simulink model "QuadSim"  (R2015a)
settings: Solver=ode45  StartTime=0.0  StopTime=10.0  RelTol=1e-3
undefined symbols (not defined in the file or in its folder): magnitude
libraries: aerolibutil x67, dspmathops x4, simulink_extras x2, dspinverses x1
(part 1 of 2)
settings Model: Creator=Nick  LastModifiedBy=Nick

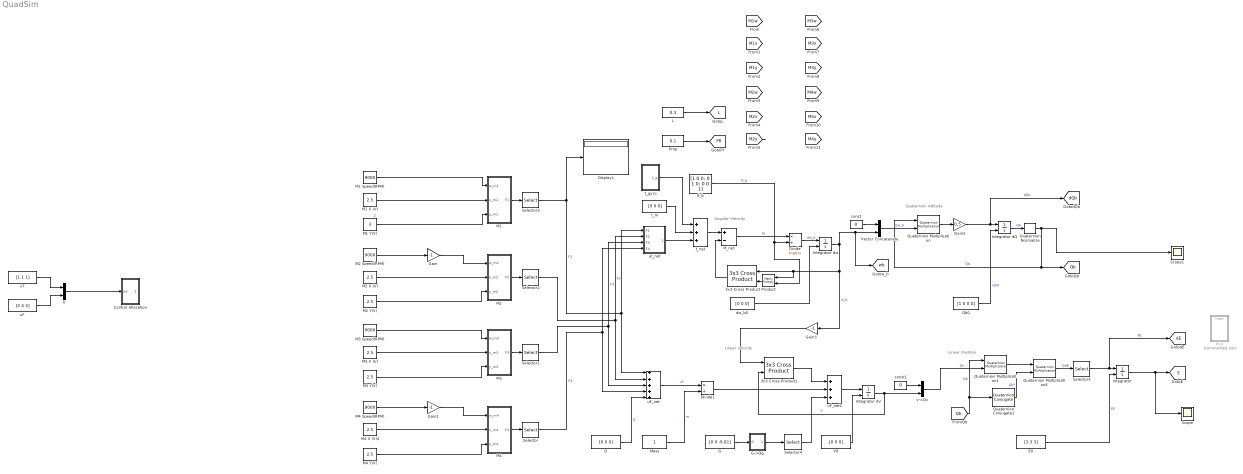
== system QuadSim ==
  note: Linear Position
  note: Linear velocity
  note: Quaternion Attitude
  note: Angular Velocity
  note: 2
  3x3 Cross Product : aerolibutil/3x3 Cross Product
  3x3 Cross Product1 : aerolibutil/3x3 Cross Product
  Control Allocation : Subsystem
  D : Constant  Value=[0 0 0]
  Display1 : Display
  Divide : Product  Inputs=*/  Multiplication=Matrix(*)
  Divide1 : Product  Inputs=*/
  E0 : Constant  Value=[3 3 3]
  G : Constant  Value=[0 0 -9.81]
  G->Qg : Subsystem
  Gain : Gain  Gain=-1
  Gain1 : Gain  Gain=-1
  Gain2 : Gain  Gain=0.5
  Gain3 : Gain  Gain=-1
  If_b : Constant  Value=[1 0 0; 0 1 0; 0 0 1]
  Integrator : Integrator  InitialConditionSource=external
  Integrator dQ : Integrator  InitialConditionSource=external  ContinuousStateAttributes='angular_acceleration'
  Integrator dV : Integrator  InitialConditionSource=external
  Integrator dw : Integrator  InitialConditionSource=external  ContinuousStateAttributes='angular_acceleration'
  L : Constant  Value=0.3
  M1 : Subsystem
  M1 Speed(RPM) : Constant  Value=9000
  M1 X (V) : Constant  Value=2.5
  M1 Y(V) : Constant  Value=3
  M2 : Subsystem
  M2 Speed(RPM) : Constant  Value=9000
  M2 X (V) : Constant  Value=2.5
  M2 Y(V) : Constant  Value=2.5
  M3 : Subsystem
  M3 Speed(RPM) : Constant  Value=9000
  M3 X (V) : Constant  Value=2.5
  M3 Y(V) : Constant  Value=2.5
  M4 : Subsystem
  M4 Speed(RPM) : Constant  Value=9000
  M4 X (V)4 : Constant  Value=2.5
  M4 Y(V) : Constant  Value=2.5
  M_net : Sum  Inputs=+-
  Mass : Constant
  Plot : Subsystem  Commented=on
  Product : Product  Multiplication=Matrix(*)
  Prop : Constant  Value=0.1
  Qb0 : Constant  Value=[1 0 0 0]
  Quaternion Conjugate1 : aerolibutil/Quaternion Conjugate
  Quaternion Multiplication : aerolibutil/Quaternion Multiplication
  Quaternion Multiplication1 : aerolibutil/Quaternion Multiplication
  Quaternion Multiplication4 : aerolibutil/Quaternion Multiplication
  Quaternion Normalize : aerolibutil/Quaternion Normalize
  Scope : Scope
      settings: YMin=0  YMax=350
  Scope1 : Scope
      settings: YMin=-1  YMax=1
  Selector{,1..5} (6 alike) : Selector  InputPortWidth=4  Indices=[2 3 4]
  U : Concatenate
  V0 : Constant  Value=[0 0 0]
  Vector Concatenate : Concatenate
  const : Constant  Value=0
  const1 : Constant  Value=0
  dw_b0 : Constant  Value=[0 0 0]
  t_gyro : Subsystem
  t_m : Constant  Value=[0 0 0]
  t_net : Sum  Inputs=+++
  uF : Constant  Value=[4 4 4]
  uF_net : Sum  Inputs=+++++
  uF_net1 : Sum  Inputs=+++
  uT : Constant  Value=[1 1 1]
  ut_net : Subsystem
  v->Qv : Concatenate
  tag scope: E=global, L=global, PR=global, Qb=global, dE=global, dQb=global, wb=global
  wires:
  M1 Speed(RPM)/1 -> M1/1(w_m1)
  M1 X (V)/1 -> M1/2(x_m1)
  M1 Y(V)/1 -> M1/3(y_m1)
  M2 X (V)/1 -> M2/2(x_m2)
  M2 Y(V)/1 -> M2/3(y_m2)
  M3 Speed(RPM)/1 -> M3/1(w_m3)
  M3 X (V)/1 -> M3/2(x_m3)
  M3 Y(V)/1 -> M3/3(y_m3)
  M4 X (V)4/1 -> M4/2(x_m4)
  M4 Y(V)/1 -> M4/3(y_m4)
  M4/1(F4) -> Selector/1
  M3/1(F3) -> Selector1/1
  M2/1(F2) -> Selector2/1
  M1/1(F1) -> Selector3/1
  Selector3/1 -> Display1/1, uF_net/1, ut_net/1(F1)  "F1"
  Selector2/1 -> ut_net/2(F2), uF_net/2  "F2"
  Selector1/1 -> uF_net/3, ut_net/3(F3)  "F3"
  Selector/1 -> ut_net/4(F4), uF_net/4  "F4"
  dw_b0/1 -> Integrator dw/2
  M_net/1 -> Divide/1  "M"
  If_b/1 -> Product/2, Divide/2  "If_b"
  Product/1 -> 3x3 Cross Product/2
  3x3 Cross Product/1 -> M_net/2
  ut_net/1(uT_diff) -> t_net/3
  t_m/1 -> t_net/2
  t_net/1 -> M_net/1
  Divide/1 -> Integrator dw/1  "dw_b"
  Integrator dw/1 -> [wb], Vector Concatenate/2, Gain3/1, Product/1, 3x3 Cross Product/1  "w_b"
  M2 Speed(RPM)/1 -> Gain/1
  Gain/1 -> M2/1(w_m2)
  M4 Speed(RPM)/1 -> Gain1/1
  Gain1/1 -> M4/1(w_m4)
  const/1 -> Vector Concatenate/1
  Vector Concatenate/1 -> Quaternion Multiplication/2  "Qw_b"
  Quaternion Multiplication/1 -> Gain2/1
  Gain2/1 -> [dQb], Integrator dQ/1  "dQb"
  Qb0/1 -> Integrator dQ/2  "Qb0"
  Quaternion Normalize/1 -> Quaternion Multiplication/1, [Qb], Scope1/1  "Qb"
  uF_net/1 -> Divide1/1  "uF"
  Mass/1 -> Divide1/2  "m"
  Divide1/1 -> uF_net1/2
  Gain3/1 -> 3x3 Cross Product1/1
  3x3 Cross Product1/1 -> uF_net1/1
  G/1 -> G->Qg/1(G)
  G->Qg/1(Qg) -> Selector4/1
  Selector4/1 -> uF_net1/3
  Integrator dQ/1 -> Quaternion Normalize/1  "Qb"
  D/1 -> uF_net/5  "D"
  uF_net1/1 -> Integrator dV/1
  V0/1 -> Integrator dV/2
  Integrator dV/1 -> 3x3 Cross Product1/2, v->Qv/2  "V"
  const1/1 -> v->Qv/1
  v->Qv/1 -> Quaternion Multiplication1/2  "Qv"
  [Qb] -> Quaternion Multiplication1/1, Quaternion Conjugate1/1  "Qb"
  Quaternion Multiplication1/1 -> Quaternion Multiplication4/1
  Quaternion Conjugate1/1 -> Quaternion Multiplication4/2  "Qb*"
  E0/1 -> Integrator/2  "E0"
  Selector5/1 -> [dE], Integrator/1  "dE"
  Quaternion Multiplication4/1 -> Selector5/1  "QdE"
  Integrator/1 -> [E], Scope/1
  [M2y] -> ?
  L/1 -> [L]
  Prop/1 -> [PR]
  uF/1 -> U/2
  uT/1 -> U/1
  t_gyro/1(t_g) -> t_net/1
  U/1 -> Control Allocation/1(Vd)

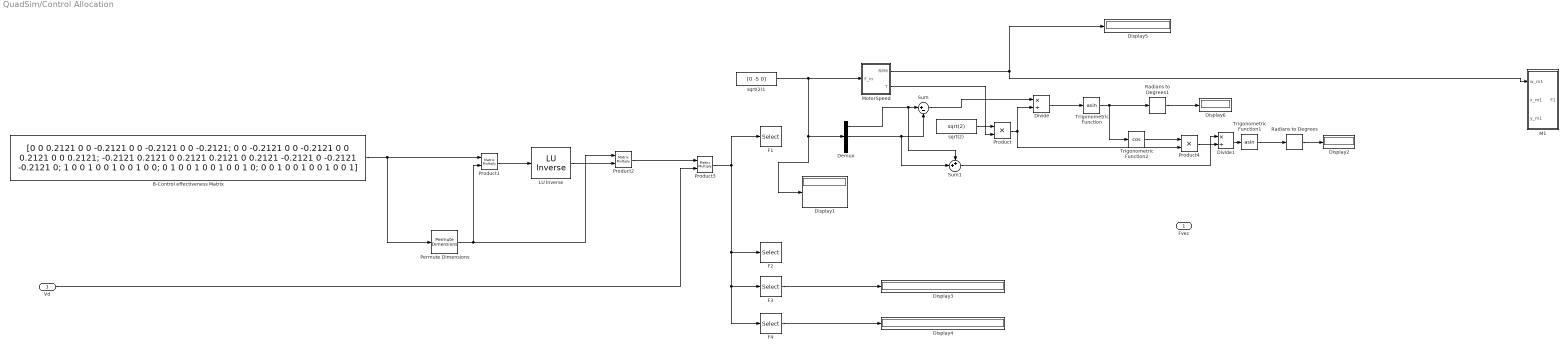
== system QuadSim/Control Allocation ==
  Vd : Inport
  " LU Inverse" : dspinverses/ LU Inverse
  B-Control effectiveness Matrix : Constant  Value=[0 0 0.2121 0 0 -0.2121 0 0 -0.2121 0 0 -0.2121; 0 0 -0.2121 0 0 -0.2121 0 0 0.2121 0 0 0.2121; -0.2121 0.2121 0 0.2121 0.2121 0 0.2121 -0.2121 0 -0.2121 -0.2121 0; 1 0 0 1 0 0 1 0 0 1 0 0; 0 1 0 0 1 0 0 1 0 0 1 0; 0 0 1 0 0 1 0 0 1 0 0 1]
  Demux : Demux  Outputs=3
  Display{1..6} (6 alike) : Display
      Display5 settings: Decimation=4
  Divide : Product  Inputs=*/
  Divide1 : Product  Inputs=*/
  F1 : Selector  InputPortWidth=12  Indices=[1 2 3]
  F2 : Selector  InputPortWidth=12  Indices=[4 5 6]
  F3 : Selector  InputPortWidth=12  Indices=[7 8 9]
  F4 : Selector  InputPortWidth=12  Indices=[10 11 12]
  M1 : Subsystem
  MotorSpeed : Subsystem
  Permute Dimensions : PermuteDimensions
  Product : Product
  Product1 : Product  Multiplication=Matrix(*)
  Product2 : Product  Multiplication=Matrix(*)
  Product3 : Product  Multiplication=Matrix(*)
  Product4 : Product
  Radians to Degrees : simulink_extras/Transformations/Radians to Degrees
  Radians to Degrees1 : simulink_extras/Transformations/Radians to Degrees
  Sum : Sum  Inputs=|+-
  Sum1 : Sum  Inputs=++|
  Trigonometric Function : Trigonometry  Operator=asin
  Trigonometric Function1 : Trigonometry  Operator=asin
  Trigonometric Function2 : Trigonometry  Operator=cos
  sqrt(2) : Constant  Value=sqrt(2)
  sqrt(2)1 : Constant  Value=[0 -5 0]
  Fvec : Outport
  wires:
  Permute Dimensions/1 -> Product1/2, Product2/1
  Product1/1 -> " LU Inverse"/1
  Product3/1 -> F1/1, F4/1, F3/1, F2/1
  Vd/1 -> Product3/2
  Product2/1 -> Product3/1
  " LU Inverse"/1 -> Product2/2
  B-Control effectiveness Matrix/1 -> Product1/1, Permute Dimensions/1
  F3/1 -> Display3/1
  F4/1 -> Display4/1
  MotorSpeed/1(RPM) -> M1/1(w_m1), Display5/1
  Demux/1 -> Sum1/1, Sum/1
  Demux/2 -> Sum1/2, Sum/2
  Product/1 -> Divide/2, Product4/2
  Sum/1 -> Divide/1
  sqrt(2)/1 -> Product/1
  Divide/1 -> Trigonometric Function/1
  Trigonometric Function/1 -> Radians to Degrees1/1, Trigonometric Function2/1
  Product4/1 -> Divide1/2
  Sum1/1 -> Divide1/1
  Divide1/1 -> Trigonometric Function1/1
  Trigonometric Function2/1 -> Product4/1
  sqrt(2)1/1 -> Display1/1, Demux/1, MotorSpeed/1(F_in)
  MotorSpeed/2(T) -> Product/2
  Trigonometric Function1/1 -> Radians to Degrees/1
  Radians to Degrees/1 -> Display2/1
  Radians to Degrees1/1 -> Display6/1

== system QuadSim/G->Qg ==
  G : Inport
  Quaternion Conjugate1 : aerolibutil/Quaternion Conjugate
  Quaternion Multiplication1 : aerolibutil/Quaternion Multiplication
  Quaternion Multiplication4 : aerolibutil/Quaternion Multiplication
  Vector Concatenate1 : Concatenate
  const1 : Constant  Value=0
  Qg : Outport
  wires:
  G/1 -> Vector Concatenate1/2
  Quaternion Multiplication1/1 -> Quaternion Multiplication4/1
  const1/1 -> Vector Concatenate1/1
  Quaternion Multiplication4/1 -> Qg/1
  [Qb] -> Quaternion Conjugate1/1, Quaternion Multiplication4/2
  Quaternion Conjugate1/1 -> Quaternion Multiplication1/1
  Vector Concatenate1/1 -> Quaternion Multiplication1/2

== system QuadSim/M1 ==
  w_m1 : Inport
  x_m1 : Inport  Port=2
  y_m1 : Inport  Port=3
  B->M1 Quaternion : Subsystem
  Const : Constant  Value=0
  F_z to Q : Concatenate  NumInputs=4
  M1 DC Motor : Subsystem
  M1 Speed to Force : Subsystem
  M1 Z(Rad) : Constant  Value=pi/4
  Quaternion Conjugate : aerolibutil/Quaternion Conjugate
  Quaternion Multiplication : aerolibutil/Quaternion Multiplication
  Quaternion Multiplication1 : aerolibutil/Quaternion Multiplication
  F1 : Outport
  tag scope: M1w=global, Qm1=global
  wires:
  Quaternion Multiplication/1 -> Quaternion Multiplication1/1
  Const/1 -> F_z to Q/1, F_z to Q/3, F_z to Q/2
  M1 DC Motor/1(Speed (rpm)) -> [M1w], M1 Speed to Force/1(Speed(RPM))
  B->M1 Quaternion/1(Q_m1) -> [Qm1], Quaternion Conjugate/1, Quaternion Multiplication/1  "Q_m1"
  w_m1/1 -> M1 DC Motor/1(Set Speed(rpm))  "w_m1"
  F_z to Q/1 -> Quaternion Multiplication/2  "Q_Fz"
  M1 Z(Rad)/1 -> B->M1 Quaternion/1("Z ")  "z_m1"
  M1 Speed to Force/1(Force(N)) -> F_z to Q/4  "F"
  y_m1/1 -> B->M1 Quaternion/3(Y)  "y_m1"
  Quaternion Conjugate/1 -> Quaternion Multiplication1/2  "Q*_m1"
  Quaternion Multiplication1/1 -> F1/1  "F_m1"
  x_m1/1 -> B->M1 Quaternion/2(X)  "x_m1"

== system QuadSim/M2 ==
  w_m2 : Inport
  x_m2 : Inport  Port=2
  y_m2 : Inport  Port=3
  B->M2 Quaternion : Subsystem
  Const : Constant  Value=0
  F_z to Q : Concatenate  NumInputs=4
  M2 DC Motor : Subsystem
  M2 Speed to Force : Subsystem
  M2 Z(Rad) : Constant  Value=3*pi/4
  Quaternion Conjugate : aerolibutil/Quaternion Conjugate
  Quaternion Multiplication : aerolibutil/Quaternion Multiplication
  Quaternion Multiplication1 : aerolibutil/Quaternion Multiplication
  F2 : Outport
  tag scope: M2w=global, Qm2=global
  wires:
  Quaternion Multiplication/1 -> Quaternion Multiplication1/1
  Quaternion Multiplication1/1 -> F2/1  "F_m2"
  Const/1 -> F_z to Q/1, F_z to Q/3, F_z to Q/2
  B->M2 Quaternion/1(Q_m2) -> [Qm2], Quaternion Conjugate/1, Quaternion Multiplication/1  "Q_m2"
  F_z to Q/1 -> Quaternion Multiplication/2  "Q_Fz"
  M2 Z(Rad)/1 -> B->M2 Quaternion/1("Z ")  "z_m1"
  x_m2/1 -> B->M2 Quaternion/2(X)  "x_m2"
  y_m2/1 -> B->M2 Quaternion/3(Y)  "y_m2"
  Quaternion Conjugate/1 -> Quaternion Multiplication1/2  "Q*_m2"
  w_m2/1 -> M2 DC Motor/1(Set Speed(rpm))  "w_m2"
  M2 DC Motor/1(Speed (rpm)) -> M2 Speed to Force/1(Speed(RPM)), [M2w]
  M2 Speed to Force/1(Force(N)) -> F_z to Q/4

== system QuadSim/M3 ==
  w_m3 : Inport
  x_m3 : Inport  Port=2
  y_m3 : Inport  Port=3
  B->M3 Quaternion : Subsystem
  Const : Constant  Value=0
  F_z to Q : Concatenate  NumInputs=4
  M3 DC Motor : Subsystem
  M3 Speed to Force : Subsystem
  M3 Z(Rad) : Constant  Value=-3*pi/4
  Quaternion Conjugate : aerolibutil/Quaternion Conjugate
  Quaternion Multiplication : aerolibutil/Quaternion Multiplication
  Quaternion Multiplication1 : aerolibutil/Quaternion Multiplication
  F3 : Outport
  tag scope: M3w=global, Qm3=global
  wires:
  Quaternion Multiplication/1 -> Quaternion Multiplication1/1
  Quaternion Multiplication1/1 -> F3/1  "F_m3"
  Const/1 -> F_z to Q/1, F_z to Q/3, F_z to Q/2
  M3 DC Motor/1(Speed (rpm)) -> M3 Speed to Force/1(Speed(RPM)), [M3w]
  B->M3 Quaternion/1(Q_m3) -> [Qm3], Quaternion Conjugate/1, Quaternion Multiplication/1  "Q_m3"
  F_z to Q/1 -> Quaternion Multiplication/2  "Q_Fz"
  M3 Z(Rad)/1 -> B->M3 Quaternion/1("Z ")  "z_m3"
  x_m3/1 -> B->M3 Quaternion/2(X)  "x_m3"
  M3 Speed to Force/1(Force(N)) -> F_z to Q/4
  y_m3/1 -> B->M3 Quaternion/3(Y)  "y_m3"
  Quaternion Conjugate/1 -> Quaternion Multiplication1/2  "Q*_m3"
  w_m3/1 -> M3 DC Motor/1(Set Speed(rpm))  "w_m3"

== system QuadSim/M4 ==
  w_m4 : Inport
  x_m4 : Inport  Port=2
  y_m4 : Inport  Port=3
  B->M4 Quaternion : Subsystem
  Const : Constant  Value=0
  F_z to Q : Concatenate  NumInputs=4
  M4 DC Motor : Subsystem
  M4 Speed to Force : Subsystem
  M4 Z(Rad) : Constant  Value=-pi/4
  Quaternion Conjugate : aerolibutil/Quaternion Conjugate
  Quaternion Multiplication : aerolibutil/Quaternion Multiplication
  Quaternion Multiplication1 : aerolibutil/Quaternion Multiplication
  F4 : Outport
  tag scope: M4w=global, Qm4=global
  wires:
  Quaternion Multiplication/1 -> Quaternion Multiplication1/1
  Quaternion Multiplication1/1 -> F4/1
  Const/1 -> F_z to Q/1, F_z to Q/3, F_z to Q/2
  M4 DC Motor/1(Speed (rpm)) -> M4 Speed to Force/1(Speed(RPM)), [M4w]
  B->M4 Quaternion/1(Q_m4) -> [Qm4], Quaternion Multiplication/1, Quaternion Conjugate/1  "Q_m4"
  w_m4/1 -> M4 DC Motor/1(Set Speed(rpm))
  F_z to Q/1 -> Quaternion Multiplication/2
  M4 Z(Rad)/1 -> B->M4 Quaternion/1("Z ")
  x_m4/1 -> B->M4 Quaternion/2(X)
  y_m4/1 -> B->M4 Quaternion/3(Y)
  Quaternion Conjugate/1 -> Quaternion Multiplication1/2
  M4 Speed to Force/1(Force(N)) -> F_z to Q/4

== system QuadSim/Plot ==
  note: Frame Plot
  Trigger : TriggerPort  PortDimensions=1
  Clock : Clock
  Plot Function : MATLAB Function  TreatAsAtomicUnit=on
  wires:
  [L] -> Plot Function/4(l)
  [PR] -> Plot Function/5(pr)
  Clock/1 -> Plot Function/3(t)
  [Qm1] -> Plot Function/6(qmtr1)
  [Qm2] -> Plot Function/7(qmtr2)
  [Qm3] -> Plot Function/8(qmtr3)
  [Qm4] -> Plot Function/9(qmtr4)
  [Qb] -> Plot Function/1(q)
  [E] -> Plot Function/2(e1)

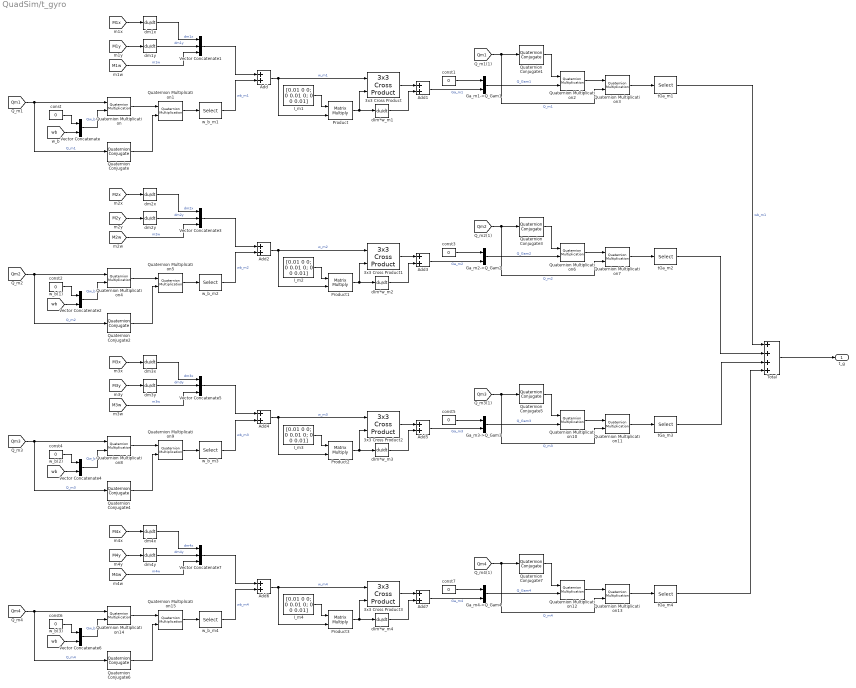
== system QuadSim/t_gyro ==
  3x3 Cross Product{,1..3} (4 alike) : aerolibutil/3x3 Cross Product
  Add{,1..7} (8 alike) : Sum
  Ga_m1->Q_Gam1 : Concatenate
  Ga_m2->Q_Gam2 : Concatenate
  Ga_m3->Q_Gam3 : Concatenate
  Ga_m4->Q_Gam4 : Concatenate
  I_m{1..4} (4 alike) : Constant  Value=[0.01 0 0; 0 0.01 0; 0 0 0.01]
  Product{,1..3} (4 alike) : Product  Multiplication=Matrix(*)
  Quaternion Conjugate{,1..7} (8 alike) : aerolibutil/Quaternion Conjugate
  Quaternion Multiplication{,1..15} (16 alike) : aerolibutil/Quaternion Multiplication
  Total : Sum  Inputs=++++
  Vector Concatenate{,2,4,6} (4 alike) : Concatenate
  Vector Concatenate{1,3,5,7} (4 alike) : Concatenate  NumInputs=3
  const{,1..7} (8 alike) : Constant  Value=0
  dIm*w_m{1..4} (4 alike) : Derivative
  dm1x : Derivative
  dm1y : Derivative
  dm2x : Derivative
  dm2y : Derivative
  dm3x : Derivative
  dm3y : Derivative
  dm4x : Derivative
  dm4y : Derivative
  tGa_m{1..4} (4 alike) : Selector  InputPortWidth=4  Indices=[2 3 4]
  w_b_m{1..4} (4 alike) : Selector  InputPortWidth=4  Indices=[2 3 4]
  t_g : Outport
  wires:
  [Qm1] -> Quaternion Conjugate/1, Quaternion Multiplication/1  "Q_m1"
  Quaternion Multiplication/1 -> Quaternion Multiplication1/1
  const/1 -> Vector Concatenate/1
  Vector Concatenate/1 -> Quaternion Multiplication/2  "Qw_b"
  [wb] -> Vector Concatenate/2
  Quaternion Multiplication1/1 -> w_b_m1/1
  [M1x] -> dm1x/1
  [M1y] -> dm1y/1
  dm1x/1 -> Vector Concatenate1/1  "dm1x"
  dm1y/1 -> Vector Concatenate1/2  "dm1y"
  [M1w] -> Vector Concatenate1/3  "m1w"
  Vector Concatenate1/1 -> Add/1
  w_b_m1/1 -> Add/2  "wb_m1"
  I_m1/1 -> Product/1
  Add/1 -> 3x3 Cross Product/1, Product/2  "w_m1"
  Product/1 -> dIm*w_m1/1, 3x3 Cross Product/2
  3x3 Cross Product/1 -> Add1/1
  dIm*w_m1/1 -> Add1/2
  Quaternion Conjugate/1 -> Quaternion Multiplication1/2
  Quaternion Multiplication3/1 -> tGa_m1/1
  const1/1 -> Ga_m1->Q_Gam1/1
  Add1/1 -> Ga_m1->Q_Gam1/2  "Ga_m1"
  Ga_m1->Q_Gam1/1 -> Quaternion Multiplication2/2  "Q_Gam1"
  Quaternion Conjugate1/1 -> Quaternion Multiplication2/1
  [Qm1] -> Quaternion Multiplication3/2, Quaternion Conjugate1/1  "Q_m1"
  Quaternion Multiplication2/1 -> Quaternion Multiplication3/1
  [Qm2] -> Quaternion Conjugate2/1, Quaternion Multiplication4/1  "Q_m2"
  Quaternion Multiplication4/1 -> Quaternion Multiplication5/1
  const2/1 -> Vector Concatenate2/1
  Vector Concatenate2/1 -> Quaternion Multiplication4/2  "Qw_b"
  [wb] -> Vector Concatenate2/2
  Quaternion Multiplication5/1 -> w_b_m2/1
  [M2x] -> dm2x/1
  [M2y] -> dm2y/1
  dm2x/1 -> Vector Concatenate3/1  "dm2x"
  dm2y/1 -> Vector Concatenate3/2  "dm2y"
  [M2w] -> Vector Concatenate3/3  "m2w"
  Vector Concatenate3/1 -> Add2/1
  w_b_m2/1 -> Add2/2  "wb_m2"
  I_m2/1 -> Product1/1
  Add2/1 -> 3x3 Cross Product1/1, Product1/2  "w_m2"
  Product1/1 -> dIm*w_m2/1, 3x3 Cross Product1/2
  3x3 Cross Product1/1 -> Add3/1
  dIm*w_m2/1 -> Add3/2
  Quaternion Conjugate2/1 -> Quaternion Multiplication5/2
  Quaternion Multiplication7/1 -> tGa_m2/1
  const3/1 -> Ga_m2->Q_Gam2/1
  Add3/1 -> Ga_m2->Q_Gam2/2  "Ga_m2"
  Ga_m2->Q_Gam2/1 -> Quaternion Multiplication6/2  "Q_Gam2"
  Quaternion Conjugate3/1 -> Quaternion Multiplication6/1
  [Qm2] -> Quaternion Multiplication7/2, Quaternion Conjugate3/1  "Q_m2"
  Quaternion Multiplication6/1 -> Quaternion Multiplication7/1
  [Qm3] -> Quaternion Conjugate4/1, Quaternion Multiplication8/1  "Q_m3"
  Quaternion Multiplication8/1 -> Quaternion Multiplication9/1
  const4/1 -> Vector Concatenate4/1
  Vector Concatenate4/1 -> Quaternion Multiplication8/2  "Qw_b"
  [wb] -> Vector Concatenate4/2
  Quaternion Multiplication9/1 -> w_b_m3/1
  [M3x] -> dm3x/1
  [M3y] -> dm3y/1
  dm3x/1 -> Vector Concatenate5/1  "dm3x"
  dm3y/1 -> Vector Concatenate5/2  "dm3y"
  [M3w] -> Vector Concatenate5/3  "m3w"
  Vector Concatenate5/1 -> Add4/1
  w_b_m3/1 -> Add4/2  "wb_m3"
  I_m3/1 -> Product2/1
  Add4/1 -> 3x3 Cross Product2/1, Product2/2  "w_m3"
  Product2/1 -> dIm*w_m3/1, 3x3 Cross Product2/2
  3x3 Cross Product2/1 -> Add5/1
  dIm*w_m3/1 -> Add5/2
  Quaternion Conjugate4/1 -> Quaternion Multiplication9/2
  Quaternion Multiplication11/1 -> tGa_m3/1
  const5/1 -> Ga_m3->Q_Gam3/1
  Add5/1 -> Ga_m3->Q_Gam3/2  "Ga_m3"
  Ga_m3->Q_Gam3/1 -> Quaternion Multiplication10/2  "Q_Gam3"
  Quaternion Conjugate5/1 -> Quaternion Multiplication10/1
  [Qm3] -> Quaternion Multiplication11/2, Quaternion Conjugate5/1  "Q_m3"
  Quaternion Multiplication10/1 -> Quaternion Multiplication11/1
  [Qm4] -> Quaternion Conjugate6/1, Quaternion Multiplication14/1  "Q_m4"
  Quaternion Multiplication14/1 -> Quaternion Multiplication15/1
  const6/1 -> Vector Concatenate6/1
  Vector Concatenate6/1 -> Quaternion Multiplication14/2  "Qw_b"
  [wb] -> Vector Concatenate6/2
  Quaternion Multiplication15/1 -> w_b_m4/1
  [M4x] -> dm4x/1
  [M4y] -> dm4y/1
  dm4x/1 -> Vector Concatenate7/1  "dm4x"
  dm4y/1 -> Vector Concatenate7/2  "dm4y"
  [M4w] -> Vector Concatenate7/3  "m4w"
  Vector Concatenate7/1 -> Add6/1
  w_b_m4/1 -> Add6/2  "wb_m4"
  I_m4/1 -> Product3/1
  Add6/1 -> 3x3 Cross Product3/1, Product3/2  "w_m4"
  Product3/1 -> dIm*w_m4/1, 3x3 Cross Product3/2
  3x3 Cross Product3/1 -> Add7/1
  dIm*w_m4/1 -> Add7/2
  Quaternion Conjugate6/1 -> Quaternion Multiplication15/2
  Quaternion Multiplication13/1 -> tGa_m4/1
  const7/1 -> Ga_m4->Q_Gam4/1
  Add7/1 -> Ga_m4->Q_Gam4/2  "Ga_m4"
  Ga_m4->Q_Gam4/1 -> Quaternion Multiplication12/2  "Q_Gam4"
  Quaternion Conjugate7/1 -> Quaternion Multiplication12/1
  [Qm4] -> Quaternion Multiplication13/2, Quaternion Conjugate7/1  "Q_m4"
  Quaternion Multiplication12/1 -> Quaternion Multiplication13/1
  tGa_m4/1 -> Total/4
  tGa_m3/1 -> Total/3
  tGa_m2/1 -> Total/2
  tGa_m1/1 -> Total/1  "wb_m1"
  Total/1 -> t_g/1

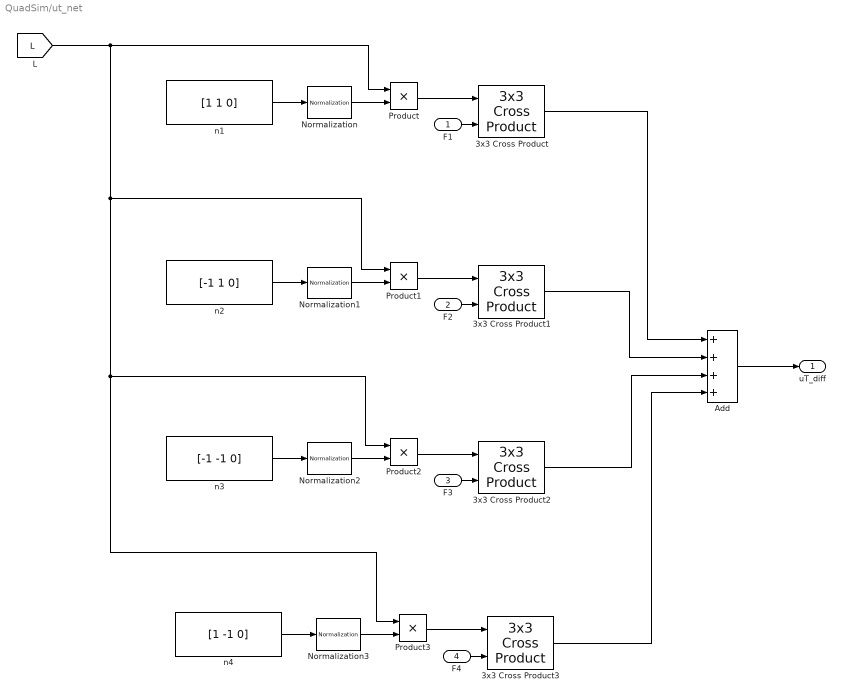
== system QuadSim/ut_net ==
  F1 : Inport
  F2 : Inport  Port=2
  F3 : Inport  Port=3
  F4 : Inport  Port=4
  3x3 Cross Product{,1..3} (4 alike) : aerolibutil/3x3 Cross Product
  Add : Sum  Inputs=++++
  Normalization{,1..3} (4 alike) : dspmathops/Normalization  NormType=2-norm  Bias=1e-10  NormOver=Each column  ColComp=off  Dimension=1  outputDataTypeStr=Inherit: Same as product output  outputLastDataTypeStr=Inherit: Same as product output  outputMin=[]  outputMax=[]  accumDataTypeStr=Inherit: Same as product output  accumLastDataTypeStr=Inherit: Same as product output  roundingMode=Floor  overflowMode=off
  Product{,1..3} (4 alike) : Product
  n1 : Constant  Value=[1 1 0]
  n2 : Constant  Value=[-1 1 0]
  n3 : Constant  Value=[-1 -1 0]
  n4 : Constant  Value=[1 -1 0]
  uT_diff : Outport
  wires:
  F1/1 -> 3x3 Cross Product/2
  Product/1 -> 3x3 Cross Product/1
  Normalization/1 -> Product/2
  3x3 Cross Product/1 -> Add/1
  n1/1 -> Normalization/1
  F2/1 -> 3x3 Cross Product1/2
  Product1/1 -> 3x3 Cross Product1/1
  Normalization1/1 -> Product1/2
  3x3 Cross Product1/1 -> Add/2
  n2/1 -> Normalization1/1
  F3/1 -> 3x3 Cross Product2/2
  Product2/1 -> 3x3 Cross Product2/1
  Normalization2/1 -> Product2/2
  3x3 Cross Product2/1 -> Add/3
  n3/1 -> Normalization2/1
  F4/1 -> 3x3 Cross Product3/2
  Product3/1 -> 3x3 Cross Product3/1
  Normalization3/1 -> Product3/2
  [L] -> Product3/1, Product2/1, Product1/1, Product/1
  3x3 Cross Product3/1 -> Add/4
  n4/1 -> Normalization3/1
  Add/1 -> uT_diff/1

== system QuadSim/Control Allocation/M1 ==
  w_m1 : Inport
  x_m1 : Inport  Port=2
  y_m1 : Inport  Port=3
  B->M1 Quaternion : Subsystem
  Const : Constant  Value=0
  F_z to Q : Concatenate  NumInputs=4
  M1 DC Motor : Subsystem
  M1 Speed to Force : Subsystem
  M1 Z(Rad) : Constant  Value=pi/4
  Quaternion Conjugate : aerolibutil/Quaternion Conjugate
  Quaternion Multiplication : aerolibutil/Quaternion Multiplication
  Quaternion Multiplication1 : aerolibutil/Quaternion Multiplication
  F1 : Outport
  wires:
  Quaternion Multiplication/1 -> Quaternion Multiplication1/1
  Const/1 -> F_z to Q/1, F_z to Q/3, F_z to Q/2
  M1 DC Motor/1(Speed (rpm)) -> M1 Speed to Force/1(Speed(RPM))
  B->M1 Quaternion/1(Q_m1) -> Quaternion Conjugate/1, Quaternion Multiplication/1  "Q_m1"
  w_m1/1 -> M1 DC Motor/1(Set Speed(rpm))  "w_m1"
  F_z to Q/1 -> Quaternion Multiplication/2  "Q_Fz"
  M1 Z(Rad)/1 -> B->M1 Quaternion/1("Z ")  "z_m1"
  M1 Speed to Force/1(Force(N)) -> F_z to Q/4  "F"
  y_m1/1 -> B->M1 Quaternion/3(Y)  "y_m1"
  Quaternion Conjugate/1 -> Quaternion Multiplication1/2  "Q*_m1"
  Quaternion Multiplication1/1 -> F1/1  "F_m1"
  x_m1/1 -> B->M1 Quaternion/2(X)  "x_m1"

== system QuadSim/Control Allocation/MotorSpeed ==
  F_in : Inport
  Divide : Product  Inputs=*/
  Force Coefficient CT : Constant  Value=0.000243
  Mins : Constant  Value=60
  Product : Product
  w^2 : Sqrt  SaturateOnIntegerOverflow=on
  |F| : Sqrt  SaturateOnIntegerOverflow=on
  |F|^2 : DotProduct  InputSameDT=on  OutDataTypeStr=Inherit: Inherit via internal rule
  RPM : Outport
  T : Outport  Port=2
  wires:
  w^2/1 -> Product/2
  Product/1 -> RPM/1  "RPM"
  Mins/1 -> Product/1
  |F|/1 -> T/1, Divide/1
  Divide/1 -> w^2/1
  Force Coefficient CT/1 -> Divide/2
  F_in/1 -> |F|^2/2, |F|^2/1
  |F|^2/1 -> |F|/1

== system QuadSim/M1/B->M1 Quaternion ==
  "Z " : Inport
  X : Inport  Port=2
  Y : Inport  Port=3
  "M1 X Servo " : Subsystem
  M1 Y Servo : Subsystem
  Quaternion Multiplication : aerolibutil/Quaternion Multiplication
  Quaternion Multiplication1 : aerolibutil/Quaternion Multiplication
  X Quaternion : Subsystem
  Y Quaternion : Subsystem
  Z Quaternion : Subsystem
  Q_m1 : Outport
  tag scope: M1x=global, M1y=global
  wires:
  X/1 -> "M1 X Servo "/1(Input(v))
  "M1 X Servo "/1(Position (rad)) -> X Quaternion/1(y(X Rad)), [M1x]
  M1 Y Servo/1(Position (rad)) -> Y Quaternion/1(h(Y Rad)), [M1y]
  "Z "/1 -> Z Quaternion/1(Z Rad)
  Z Quaternion/1(Q_z) -> Quaternion Multiplication/1  "Qz"
  Quaternion Multiplication/1 -> Quaternion Multiplication1/1  "Qz*Qy"
  Quaternion Multiplication1/1 -> Q_m1/1  "Qz*Qy*Qx"
  Y/1 -> M1 Y Servo/1(Input(v))
  Y Quaternion/1(Q_y) -> Quaternion Multiplication/2  "Qy"
  X Quaternion/1(Q_x) -> Quaternion Multiplication1/2

== system QuadSim/M1/M1 DC Motor ==
  note: M1 DC Motor response
  Set Speed(rpm) : Inport
  ->ms : Product  Inputs=*/
  10080 Max : Saturate  UpperLimit=10080  LowerLimit=-10080
  Add : Sum
  Dead Time (ms) : Constant
  Dead Time Block : VariableTransportDelay  MaximumDelay=10
  Miliseconds : Constant  Value=1000
  Starting Speed : Constant  Value=10080
  Subtract : Sum  Inputs=+-
  Transfer Fcn : TransferFcn  Numerator=1  Denominator=[0.6 1]
  Speed (rpm) : Outport
  wires:
  Dead Time Block/1 -> Transfer Fcn/1
  Miliseconds/1 -> ->ms/2
  Dead Time (ms)/1 -> ->ms/1
  ->ms/1 -> Dead Time Block/2
  Transfer Fcn/1 -> 10080 Max/1
  Set Speed(rpm)/1 -> Subtract/1
  10080 Max/1 -> Add/1
  Add/1 -> Speed (rpm)/1
  Starting Speed/1 -> Subtract/2, Add/2
  Subtract/1 -> Dead Time Block/1

== system QuadSim/M1/M1 Speed to Force ==
  note: RPS to Force
  Speed(RPM) : Inport
  ->RPS : Product  Inputs=*/
  Force Coefficient CT : Constant  Value=0.000243
  M1 w^2 : Math  Operator=magnitude^2  SaturateOnIntegerOverflow=on
  Mins : Constant  Value=60
  Product : Product
  Force(N) : Outport
  wires:
  M1 w^2/1 -> Product/2
  ->RPS/1 -> M1 w^2/1
  Speed(RPM)/1 -> ->RPS/1
  Force Coefficient CT/1 -> Product/1
  Mins/1 -> ->RPS/2
  Product/1 -> Force(N)/1

== system QuadSim/M2/B->M2 Quaternion ==
  "Z " : Inport
  X : Inport  Port=2
  Y : Inport  Port=3
  "M2 X Servo " : Subsystem
  "M2 Y Servo " : Subsystem
  Quaternion Multiplication : aerolibutil/Quaternion Multiplication
  Quaternion Multiplication1 : aerolibutil/Quaternion Multiplication
  X Quaternion : Subsystem
  Y Quaternion : Subsystem
  Z Quaternion : Subsystem
  Q_m2 : Outport
  tag scope: M2x=global, M2y=global
  wires:
  X/1 -> "M2 X Servo "/1(Input(v))
  Y/1 -> "M2 Y Servo "/1(Input(v))
  "M2 X Servo "/1(Position (rad)) -> [M2x], X Quaternion/1(y(X Rad))
  "M2 Y Servo "/1(Position (rad)) -> [M2y], Y Quaternion/1(h(Y Rad))
  "Z "/1 -> Z Quaternion/1(Z Rad)
  Z Quaternion/1(Q_z) -> Quaternion Multiplication/1  "Qz"
  Quaternion Multiplication/1 -> Quaternion Multiplication1/1  "Qz*Qy"
  Quaternion Multiplication1/1 -> Q_m2/1  "Qz*Qy*Qx"
  X Quaternion/1(Q_x) -> Quaternion Multiplication1/2  "Qx"
  Y Quaternion/1(Q_y) -> Quaternion Multiplication/2  "Qy"

== system QuadSim/M2/M2 DC Motor ==
  note: M2 DC Motor response
  Set Speed(rpm) : Inport
  ->ms : Product  Inputs=*/
  10080 Max : Saturate  UpperLimit=10080  LowerLimit=0
  Add : Sum
  Dead Time (ms) : Constant
  Dead Time Block : VariableTransportDelay  MaximumDelay=10
  Gain : Gain  Gain=-1
  Miliseconds : Constant  Value=1000
  Starting Speed : Constant  Value=10080
  Subtract : Sum  Inputs=+-
  Transfer Fcn : TransferFcn  Numerator=1  Denominator=[0.6 1]
  Speed (rpm) : Outport
  wires:
  Dead Time Block/1 -> Transfer Fcn/1
  Miliseconds/1 -> ->ms/2
  Dead Time (ms)/1 -> ->ms/1
  ->ms/1 -> Dead Time Block/2
  Transfer Fcn/1 -> 10080 Max/1
  Set Speed(rpm)/1 -> Subtract/1
  10080 Max/1 -> Add/1
  Add/1 -> Speed (rpm)/1
  Gain/1 -> Subtract/2, Add/2
  Starting Speed/1 -> Gain/1
  Subtract/1 -> Dead Time Block/1

== system QuadSim/M2/M2 Speed to Force ==
  note: RPS to Force
  Speed(RPM) : Inport
  ->RPS : Product  Inputs=*/
  Abs : Abs
  Force Coefficient CT : Constant  Value=0.000243
  M2 w^2 : Math  Operator=magnitude^2  SaturateOnIntegerOverflow=on
  Mins : Constant  Value=60
  Product : Product
  Force(N) : Outport
  wires:
  M2 w^2/1 -> Product/2
  ->RPS/1 -> M2 w^2/1
  Force Coefficient CT/1 -> Product/1
  Mins/1 -> ->RPS/2
  Product/1 -> Force(N)/1
  Abs/1 -> ->RPS/1
  Speed(RPM)/1 -> Abs/1

== system QuadSim/M3/B->M3 Quaternion ==
  "Z " : Inport
  X : Inport  Port=2
  Y : Inport  Port=3
  "M3 X Servo " : Subsystem
  "M3\\ Y Servo " : Subsystem
  Quaternion Multiplication : aerolibutil/Quaternion Multiplication
  Quaternion Multiplication1 : aerolibutil/Quaternion Multiplication
  X Quaternion : Subsystem
  Y Quaternion : Subsystem
  Z Quaternion : Subsystem
  Q_m3 : Outport
  tag scope: M3x=global, M3y=global
  wires:
  X/1 -> "M3 X Servo "/1(Input(v))
  Y/1 -> "M3\\ Y Servo "/1(Input(v))
  "M3 X Servo "/1(Position (rad)) -> [M3x], X Quaternion/1(y(X Rad))
  "M3\\ Y Servo "/1(Position (rad)) -> [M3y], Y Quaternion/1(h(Y Rad))
  "Z "/1 -> Z Quaternion/1(Z Rad)
  Z Quaternion/1(Q_z) -> Quaternion Multiplication/1  "Qz"
  Quaternion Multiplication/1 -> Quaternion Multiplication1/1  "Qz*Qy"
  Quaternion Multiplication1/1 -> Q_m3/1  "Qz*Qy*Qx"
  X Quaternion/1(Q_x) -> Quaternion Multiplication1/2  "Qx"
  Y Quaternion/1(Q_y) -> Quaternion Multiplication/2  "Qy"

== system QuadSim/M3/M3 DC Motor ==
  note: M3 DC Motor response
  Set Speed(rpm) : Inport
  ->ms : Product  Inputs=*/
  10080 Max : Saturate  UpperLimit=10080  LowerLimit=-10080
  Add : Sum
  Dead Time (ms) : Constant
  Dead Time Block : VariableTransportDelay  MaximumDelay=10
  Miliseconds : Constant  Value=1000
  Starting Speed : Constant  Value=10080
  Subtract : Sum  Inputs=+-
  Transfer Fcn : TransferFcn  Numerator=1  Denominator=[0.6 1]
  Speed (rpm) : Outport
  wires:
  Dead Time Block/1 -> Transfer Fcn/1
  Miliseconds/1 -> ->ms/2
  Dead Time (ms)/1 -> ->ms/1
  ->ms/1 -> Dead Time Block/2
  Transfer Fcn/1 -> 10080 Max/1
  Subtract/1 -> Dead Time Block/1
  Set Speed(rpm)/1 -> Subtract/1
  10080 Max/1 -> Add/1
  Add/1 -> Speed (rpm)/1
  Starting Speed/1 -> Subtract/2, Add/2

== system QuadSim/M3/M3 Speed to Force ==
  note: RPS to Force
  Speed(RPM) : Inport
  ->RPS : Product  Inputs=*/
  Abs : Abs
  Force Coefficient CT : Constant  Value=0.000243
  M3 w^2 : Math  Operator=magnitude^2  SaturateOnIntegerOverflow=on
  Mins : Constant  Value=60
  Product : Product
  Force(N) : Outport
  wires:
  M3 w^2/1 -> Product/2
  ->RPS/1 -> M3 w^2/1
  Force Coefficient CT/1 -> Product/1
  Mins/1 -> ->RPS/2
  Product/1 -> Force(N)/1
  Abs/1 -> ->RPS/1
  Speed(RPM)/1 -> Abs/1

== system QuadSim/M4/B->M4 Quaternion ==
  "Z " : Inport
  X : Inport  Port=2
  Y : Inport  Port=3
  "M4 X Servo " : Subsystem
  "M4 Y Servo " : Subsystem
  Quaternion Multiplication : aerolibutil/Quaternion Multiplication
  Quaternion Multiplication1 : aerolibutil/Quaternion Multiplication
  X Quaternion : Subsystem
  Y Quaternion : Subsystem
  Z Quaternion : Subsystem
  Q_m4 : Outport
  tag scope: M4x=global, M4y=global
  wires:
  X/1 -> "M4 X Servo "/1(Input(v))
  Y/1 -> "M4 Y Servo "/1(Input(v))
  "M4 X Servo "/1(Position (rad)) -> [M4x], X Quaternion/1(y(X Rad))
  "M4 Y Servo "/1(Position (rad)) -> [M4y], Y Quaternion/1(h(Y Rad))
  "Z "/1 -> Z Quaternion/1(Z Rad)
  Z Quaternion/1(Q_z) -> Quaternion Multiplication/1  "Qz"
  Quaternion Multiplication/1 -> Quaternion Multiplication1/1  "Qz*Qy"
  Quaternion Multiplication1/1 -> Q_m4/1  "Qz*Qy*Qx"
  X Quaternion/1(Q_x) -> Quaternion Multiplication1/2  "Qx"
  Y Quaternion/1(Q_y) -> Quaternion Multiplication/2  "Qy"

== system QuadSim/M4/M4 DC Motor ==
  note: M4 DC Motor response
  Set Speed(rpm) : Inport
  ->ms : Product  Inputs=*/
  10080 Max : Saturate  UpperLimit=10080  LowerLimit=-10080
  Add : Sum
  Dead Time (ms) : Constant
  Dead Time Block : VariableTransportDelay  MaximumDelay=10
  Gain : Gain  Gain=-1
  Miliseconds : Constant  Value=1000
  Starting Speed : Constant  Value=10080
  Subtract : Sum  Inputs=+-
  Transfer Fcn : TransferFcn  Numerator=1  Denominator=[0.6 1]
  Speed (rpm) : Outport
  wires:
  Dead Time Block/1 -> Transfer Fcn/1
  Miliseconds/1 -> ->ms/2
  Dead Time (ms)/1 -> ->ms/1
  ->ms/1 -> Dead Time Block/2
  Transfer Fcn/1 -> 10080 Max/1
  Subtract/1 -> Dead Time Block/1
  Set Speed(rpm)/1 -> Subtract/1
  10080 Max/1 -> Add/1
  Add/1 -> Speed (rpm)/1
  Gain/1 -> Subtract/2, Add/2
  Starting Speed/1 -> Gain/1

== system QuadSim/M4/M4 Speed to Force ==
  note: RPS to Force
  Speed(RPM) : Inport
  ->RPS : Product  Inputs=*/
  Abs : Abs
  Force Coefficient CT : Constant  Value=0.000243
  M4 w^2 : Math  Operator=magnitude^2  SaturateOnIntegerOverflow=on
  Mins : Constant  Value=60
  Product : Product
  Force(N) : Outport
  wires:
  M4 w^2/1 -> Product/2
  ->RPS/1 -> M4 w^2/1
  Force Coefficient CT/1 -> Product/1
  Mins/1 -> ->RPS/2
  Product/1 -> Force(N)/1
  Abs/1 -> ->RPS/1
  Speed(RPM)/1 -> Abs/1

== system QuadSim/Control Allocation/M1/B->M1 Quaternion ==
  "Z " : Inport
  X : Inport  Port=2
  Y : Inport  Port=3
  "M1 X Servo " : Subsystem
  M1 Y Servo : Subsystem
  Quaternion Multiplication : aerolibutil/Quaternion Multiplication
  Quaternion Multiplication1 : aerolibutil/Quaternion Multiplication
  X Quaternion : Subsystem
  Y Quaternion : Subsystem
  Z Quaternion : Subsystem
  Q_m1 : Outport
  wires:
  X/1 -> "M1 X Servo "/1(Input(v))
  "M1 X Servo "/1(Position (rad)) -> X Quaternion/1(y(X Rad))
  M1 Y Servo/1(Position (rad)) -> Y Quaternion/1(h(Y Rad))
  "Z "/1 -> Z Quaternion/1(Z Rad)
  Z Quaternion/1(Q_z) -> Quaternion Multiplication/1  "Qz"
  Quaternion Multiplication/1 -> Quaternion Multiplication1/1  "Qz*Qy"
  Quaternion Multiplication1/1 -> Q_m1/1  "Qz*Qy*Qx"
  Y/1 -> M1 Y Servo/1(Input(v))
  Y Quaternion/1(Q_y) -> Quaternion Multiplication/2  "Qy"
  X Quaternion/1(Q_x) -> Quaternion Multiplication1/2

== system QuadSim/Control Allocation/M1/M1 DC Motor ==
  note: M1 DC Motor response
  Set Speed(rpm) : Inport
  ->ms : Product  Inputs=*/
  10080 Max : Saturate  UpperLimit=10080  LowerLimit=-10080
  Add : Sum
  Dead Time (ms) : Constant
  Dead Time Block : VariableTransportDelay  MaximumDelay=10
  Miliseconds : Constant  Value=1000
  Starting Speed : Constant  Value=10080
  Subtract : Sum  Inputs=+-
  Transfer Fcn : TransferFcn  Numerator=1  Denominator=[0.6 1]
  Speed (rpm) : Outport
  wires:
  Dead Time Block/1 -> Transfer Fcn/1
  Miliseconds/1 -> ->ms/2
  Dead Time (ms)/1 -> ->ms/1
  ->ms/1 -> Dead Time Block/2
  Transfer Fcn/1 -> 10080 Max/1
  Set Speed(rpm)/1 -> Subtract/1
  10080 Max/1 -> Add/1
  Add/1 -> Speed (rpm)/1
  Starting Speed/1 -> Subtract/2, Add/2
  Subtract/1 -> Dead Time Block/1

== system QuadSim/Control Allocation/M1/M1 Speed to Force ==
  note: RPS to Force
  Speed(RPM) : Inport
  ->RPS : Product  Inputs=*/
  Force Coefficient CT : Constant  Value=0.000243
  M1 w^2 : Math  Operator=magnitude^2  SaturateOnIntegerOverflow=on
  Mins : Constant  Value=60
  Product : Product
  Force(N) : Outport
  wires:
  M1 w^2/1 -> Product/2
  ->RPS/1 -> M1 w^2/1
  Speed(RPM)/1 -> ->RPS/1
  Force Coefficient CT/1 -> Product/1
  Mins/1 -> ->RPS/2
  Product/1 -> Force(N)/1

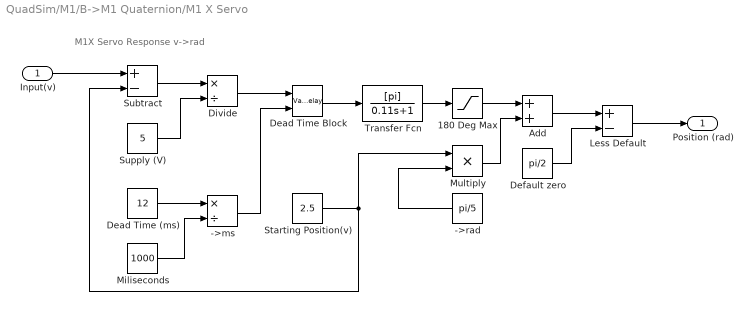
== system QuadSim/M1/B->M1 Quaternion/M1 X Servo  ==
  note: M1X Servo Response v->rad
  Input(v) : Inport
  ->ms : Product  Inputs=*/
  ->rad : Constant  Value=pi/5
  180 Deg Max : Saturate  UpperLimit=pi/2  LowerLimit=-pi/2
  Add : Sum
  Dead Time (ms) : Constant  Value=12
  Dead Time Block : VariableTransportDelay  MaximumDelay=10
  Default zero : Constant  Value=pi/2
  Divide : Product  Inputs=*/
  Less Default : Sum  Inputs=+-
  Miliseconds : Constant  Value=1000
  Multiply : Product  Inputs=**
  Starting Position(v) : Constant  Value=2.5
  Subtract : Sum  Inputs=+-
  Supply (V) : Constant  Value=5
  Transfer Fcn : TransferFcn  Numerator=[pi]  Denominator=[0.11 1]
  Position (rad) : Outport
  wires:
  Miliseconds/1 -> ->ms/2
  Dead Time (ms)/1 -> ->ms/1
  Default zero/1 -> Less Default/2
  Starting Position(v)/1 -> Multiply/1, Subtract/2
  Subtract/1 -> Divide/1
  Supply (V)/1 -> Divide/2
  Divide/1 -> Dead Time Block/1
  ->ms/1 -> Dead Time Block/2
  Dead Time Block/1 -> Transfer Fcn/1
  Transfer Fcn/1 -> 180 Deg Max/1
  180 Deg Max/1 -> Add/1
  ->rad/1 -> Multiply/2
  Multiply/1 -> Add/2
  Less Default/1 -> Position (rad)/1
  Add/1 -> Less Default/1
  Input(v)/1 -> Subtract/1

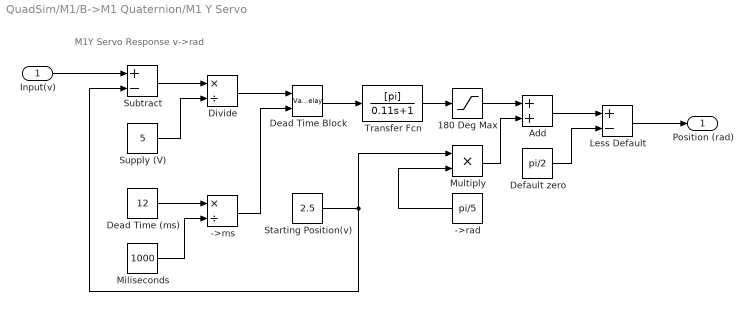
== system QuadSim/M1/B->M1 Quaternion/M1 Y Servo ==
  note: M1Y Servo Response v->rad
  Input(v) : Inport
  ->ms : Product  Inputs=*/
  ->rad : Constant  Value=pi/5
  180 Deg Max : Saturate  UpperLimit=pi/2  LowerLimit=-pi/2
  Add : Sum
  Dead Time (ms) : Constant  Value=12
  Dead Time Block : VariableTransportDelay  MaximumDelay=10
  Default zero : Constant  Value=pi/2
  Divide : Product  Inputs=*/
  Less Default : Sum  Inputs=+-
  Miliseconds : Constant  Value=1000
  Multiply : Product  Inputs=**
  Starting Position(v) : Constant  Value=2.5
  Subtract : Sum  Inputs=+-
  Supply (V) : Constant  Value=5
  Transfer Fcn : TransferFcn  Numerator=[pi]  Denominator=[0.11 1]
  Position (rad) : Outport
  wires:
  Miliseconds/1 -> ->ms/2
  Dead Time (ms)/1 -> ->ms/1
  Default zero/1 -> Less Default/2
  Starting Position(v)/1 -> Multiply/1, Subtract/2
  Subtract/1 -> Divide/1
  Supply (V)/1 -> Divide/2
  Divide/1 -> Dead Time Block/1
  ->ms/1 -> Dead Time Block/2
  Dead Time Block/1 -> Transfer Fcn/1
  Transfer Fcn/1 -> 180 Deg Max/1
  180 Deg Max/1 -> Add/1
  ->rad/1 -> Multiply/2
  Multiply/1 -> Add/2
  Less Default/1 -> Position (rad)/1
  Add/1 -> Less Default/1
  Input(v)/1 -> Subtract/1

== system QuadSim/M1/B->M1 Quaternion/X Quaternion ==
  y(X Rad) : Inport
  Const : Constant  Value=2
  Const1 : Constant  Value=0
  Divide : Product  Inputs=*/
  Trigonometric Function : Trigonometry  Operator=cos
  Trigonometric Function1 : Trigonometry
  Vector Concatenate : Concatenate  NumInputs=4
  Q_x : Outport
  wires:
  Vector Concatenate/1 -> Q_x/1
  Const/1 -> Divide/2
  Trigonometric Function1/1 -> Vector Concatenate/2
  Trigonometric Function/1 -> Vector Concatenate/1
  Const1/1 -> Vector Concatenate/4, Vector Concatenate/3
  Divide/1 -> Trigonometric Function1/1, Trigonometric Function/1
  y(X Rad)/1 -> Divide/1

== system QuadSim/M1/B->M1 Quaternion/Y Quaternion ==
  h(Y Rad) : Inport
  Const : Constant  Value=2
  Const1 : Constant  Value=0
  Divide : Product  Inputs=*/
  Trigonometric Function : Trigonometry  Operator=cos
  Trigonometric Function1 : Trigonometry
  Vector Concatenate : Concatenate  NumInputs=4
  Q_y : Outport
  wires:
  Vector Concatenate/1 -> Q_y/1
  Const/1 -> Divide/2
  Trigonometric Function/1 -> Vector Concatenate/1
  Const1/1 -> Vector Concatenate/2, Vector Concatenate/4
  Divide/1 -> Trigonometric Function1/1, Trigonometric Function/1
  h(Y Rad)/1 -> Divide/1
  Trigonometric Function1/1 -> Vector Concatenate/3

== system QuadSim/M1/B->M1 Quaternion/Z Quaternion ==
  Z Rad : Inport
  Const : Constant  Value=2
  Const1 : Constant  Value=0
  Divide : Product  Inputs=*/
  Trigonometric Function : Trigonometry  Operator=cos
  Trigonometric Function1 : Trigonometry
  Vector Concatenate : Concatenate  NumInputs=4
  Q_z : Outport
  wires:
  Vector Concatenate/1 -> Q_z/1
  Const/1 -> Divide/2
  Trigonometric Function/1 -> Vector Concatenate/1
  Const1/1 -> Vector Concatenate/3, Vector Concatenate/2
  Divide/1 -> Trigonometric Function1/1, Trigonometric Function/1
  Z Rad/1 -> Divide/1
  Trigonometric Function1/1 -> Vector Concatenate/4

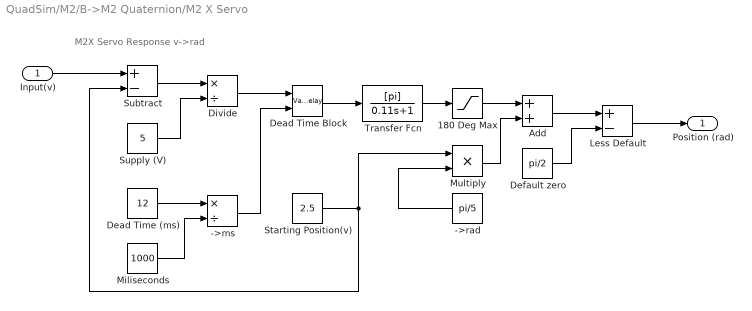
== system QuadSim/M2/B->M2 Quaternion/M2 X Servo  ==
  note: M2X Servo Response v->rad
  Input(v) : Inport
  ->ms : Product  Inputs=*/
  ->rad : Constant  Value=pi/5
  180 Deg Max : Saturate  UpperLimit=pi/2  LowerLimit=-pi/2
  Add : Sum
  Dead Time (ms) : Constant  Value=12
  Dead Time Block : VariableTransportDelay  MaximumDelay=10
  Default zero : Constant  Value=pi/2
  Divide : Product  Inputs=*/
  Less Default : Sum  Inputs=+-
  Miliseconds : Constant  Value=1000
  Multiply : Product  Inputs=**
  Starting Position(v) : Constant  Value=2.5
  Subtract : Sum  Inputs=+-
  Supply (V) : Constant  Value=5
  Transfer Fcn : TransferFcn  Numerator=[pi]  Denominator=[0.11 1]
  Position (rad) : Outport
  wires:
  Miliseconds/1 -> ->ms/2
  Dead Time (ms)/1 -> ->ms/1
  Default zero/1 -> Less Default/2
  Starting Position(v)/1 -> Multiply/1, Subtract/2
  Subtract/1 -> Divide/1
  Supply (V)/1 -> Divide/2
  Divide/1 -> Dead Time Block/1
  ->ms/1 -> Dead Time Block/2
  Dead Time Block/1 -> Transfer Fcn/1
  Transfer Fcn/1 -> 180 Deg Max/1
  180 Deg Max/1 -> Add/1
  ->rad/1 -> Multiply/2
  Multiply/1 -> Add/2
  Less Default/1 -> Position (rad)/1
  Add/1 -> Less Default/1
  Input(v)/1 -> Subtract/1

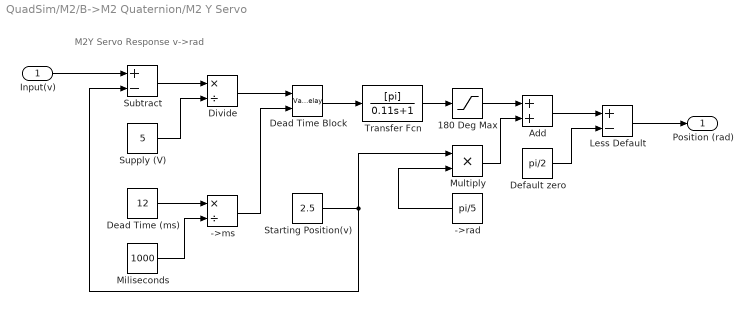
== system QuadSim/M2/B->M2 Quaternion/M2 Y Servo  ==
  note: M2Y Servo Response v->rad
  Input(v) : Inport
  ->ms : Product  Inputs=*/
  ->rad : Constant  Value=pi/5
  180 Deg Max : Saturate  UpperLimit=pi/2  LowerLimit=-pi/2
  Add : Sum
  Dead Time (ms) : Constant  Value=12
  Dead Time Block : VariableTransportDelay  MaximumDelay=10
  Default zero : Constant  Value=pi/2
  Divide : Product  Inputs=*/
  Less Default : Sum  Inputs=+-
  Miliseconds : Constant  Value=1000
  Multiply : Product  Inputs=**
  Starting Position(v) : Constant  Value=2.5
  Subtract : Sum  Inputs=+-
  Supply (V) : Constant  Value=5
  Transfer Fcn : TransferFcn  Numerator=[pi]  Denominator=[0.11 1]
  Position (rad) : Outport
  wires:
  Miliseconds/1 -> ->ms/2
  Dead Time (ms)/1 -> ->ms/1
  Default zero/1 -> Less Default/2
  Starting Position(v)/1 -> Multiply/1, Subtract/2
  Subtract/1 -> Divide/1
  Supply (V)/1 -> Divide/2
  Divide/1 -> Dead Time Block/1
  ->ms/1 -> Dead Time Block/2
  Dead Time Block/1 -> Transfer Fcn/1
  Transfer Fcn/1 -> 180 Deg Max/1
  180 Deg Max/1 -> Add/1
  ->rad/1 -> Multiply/2
  Multiply/1 -> Add/2
  Less Default/1 -> Position (rad)/1
  Add/1 -> Less Default/1
  Input(v)/1 -> Subtract/1

== system QuadSim/M2/B->M2 Quaternion/X Quaternion ==
  y(X Rad) : Inport
  Const : Constant  Value=2
  Const1 : Constant  Value=0
  Divide : Product  Inputs=*/
  Trigonometric Function : Trigonometry  Operator=cos
  Trigonometric Function1 : Trigonometry
  Vector Concatenate : Concatenate  NumInputs=4
  Q_x : Outport
  wires:
  Vector Concatenate/1 -> Q_x/1
  Const/1 -> Divide/2
  Trigonometric Function1/1 -> Vector Concatenate/2
  Trigonometric Function/1 -> Vector Concatenate/1
  Const1/1 -> Vector Concatenate/4, Vector Concatenate/3
  Divide/1 -> Trigonometric Function1/1, Trigonometric Function/1
  y(X Rad)/1 -> Divide/1

== system QuadSim/M2/B->M2 Quaternion/Y Quaternion ==
  h(Y Rad) : Inport
  Const : Constant  Value=2
  Const1 : Constant  Value=0
  Divide : Product  Inputs=*/
  Trigonometric Function : Trigonometry  Operator=cos
  Trigonometric Function1 : Trigonometry
  Vector Concatenate : Concatenate  NumInputs=4
  Q_y : Outport
  wires:
  Vector Concatenate/1 -> Q_y/1
  Const/1 -> Divide/2
  Trigonometric Function/1 -> Vector Concatenate/1
  Const1/1 -> Vector Concatenate/2, Vector Concatenate/4
  Divide/1 -> Trigonometric Function1/1, Trigonometric Function/1
  h(Y Rad)/1 -> Divide/1
  Trigonometric Function1/1 -> Vector Concatenate/3

== system QuadSim/M2/B->M2 Quaternion/Z Quaternion ==
  Z Rad : Inport
  Const : Constant  Value=2
  Const1 : Constant  Value=0
  Divide : Product  Inputs=*/
  Trigonometric Function : Trigonometry  Operator=cos
  Trigonometric Function1 : Trigonometry
  Vector Concatenate : Concatenate  NumInputs=4
  Q_z : Outport
  wires:
  Vector Concatenate/1 -> Q_z/1
  Const/1 -> Divide/2
  Trigonometric Function/1 -> Vector Concatenate/1
  Const1/1 -> Vector Concatenate/3, Vector Concatenate/2
  Divide/1 -> Trigonometric Function1/1, Trigonometric Function/1
  Z Rad/1 -> Divide/1
  Trigonometric Function1/1 -> Vector Concatenate/4

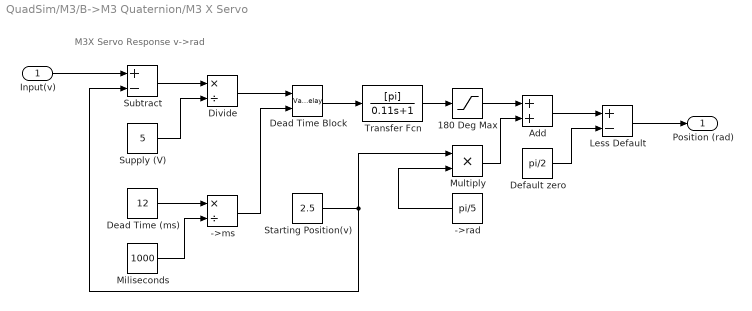
== system QuadSim/M3/B->M3 Quaternion/M3 X Servo  ==
  note: M3X Servo Response v->rad
  Input(v) : Inport
  ->ms : Product  Inputs=*/
  ->rad : Constant  Value=pi/5
  180 Deg Max : Saturate  UpperLimit=pi/2  LowerLimit=-pi/2
  Add : Sum
  Dead Time (ms) : Constant  Value=12
  Dead Time Block : VariableTransportDelay  MaximumDelay=10
  Default zero : Constant  Value=pi/2
  Divide : Product  Inputs=*/
  Less Default : Sum  Inputs=+-
  Miliseconds : Constant  Value=1000
  Multiply : Product  Inputs=**
  Starting Position(v) : Constant  Value=2.5
  Subtract : Sum  Inputs=+-
  Supply (V) : Constant  Value=5
  Transfer Fcn : TransferFcn  Numerator=[pi]  Denominator=[0.11 1]
  Position (rad) : Outport
  wires:
  Miliseconds/1 -> ->ms/2
  Dead Time (ms)/1 -> ->ms/1
  Default zero/1 -> Less Default/2
  Starting Position(v)/1 -> Multiply/1, Subtract/2
  Subtract/1 -> Divide/1
  Supply (V)/1 -> Divide/2
  Divide/1 -> Dead Time Block/1
  ->ms/1 -> Dead Time Block/2
  Dead Time Block/1 -> Transfer Fcn/1
  Transfer Fcn/1 -> 180 Deg Max/1
  180 Deg Max/1 -> Add/1
  ->rad/1 -> Multiply/2
  Multiply/1 -> Add/2
  Less Default/1 -> Position (rad)/1
  Add/1 -> Less Default/1
  Input(v)/1 -> Subtract/1

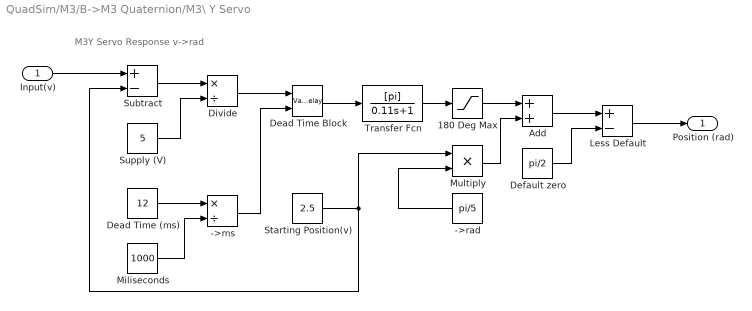
== system QuadSim/M3/B->M3 Quaternion/M3\ Y Servo  ==
  note: M3Y Servo Response v->rad
  Input(v) : Inport
  ->ms : Product  Inputs=*/
  ->rad : Constant  Value=pi/5
  180 Deg Max : Saturate  UpperLimit=pi/2  LowerLimit=-pi/2
  Add : Sum
  Dead Time (ms) : Constant  Value=12
  Dead Time Block : VariableTransportDelay  MaximumDelay=10
  Default zero : Constant  Value=pi/2
  Divide : Product  Inputs=*/
  Less Default : Sum  Inputs=+-
  Miliseconds : Constant  Value=1000
  Multiply : Product  Inputs=**
  Starting Position(v) : Constant  Value=2.5
  Subtract : Sum  Inputs=+-
  Supply (V) : Constant  Value=5
  Transfer Fcn : TransferFcn  Numerator=[pi]  Denominator=[0.11 1]
  Position (rad) : Outport
  wires:
  Miliseconds/1 -> ->ms/2
  Dead Time (ms)/1 -> ->ms/1
  Default zero/1 -> Less Default/2
  Starting Position(v)/1 -> Multiply/1, Subtract/2
  Subtract/1 -> Divide/1
  Supply (V)/1 -> Divide/2
  Divide/1 -> Dead Time Block/1
  ->ms/1 -> Dead Time Block/2
  Dead Time Block/1 -> Transfer Fcn/1
  Transfer Fcn/1 -> 180 Deg Max/1
  180 Deg Max/1 -> Add/1
  ->rad/1 -> Multiply/2
  Multiply/1 -> Add/2
  Less Default/1 -> Position (rad)/1
  Add/1 -> Less Default/1
  Input(v)/1 -> Subtract/1

== system QuadSim/M3/B->M3 Quaternion/X Quaternion ==
  y(X Rad) : Inport
  Const : Constant  Value=2
  Const1 : Constant  Value=0
  Divide : Product  Inputs=*/
  Trigonometric Function : Trigonometry  Operator=cos
  Trigonometric Function1 : Trigonometry
  Vector Concatenate : Concatenate  NumInputs=4
  Q_x : Outport
  wires:
  Vector Concatenate/1 -> Q_x/1
  Const/1 -> Divide/2
  Trigonometric Function1/1 -> Vector Concatenate/2
  Trigonometric Function/1 -> Vector Concatenate/1
  Const1/1 -> Vector Concatenate/4, Vector Concatenate/3
  Divide/1 -> Trigonometric Function1/1, Trigonometric Function/1
  y(X Rad)/1 -> Divide/1

== system QuadSim/M3/B->M3 Quaternion/Y Quaternion ==
  h(Y Rad) : Inport
  Const : Constant  Value=2
  Const1 : Constant  Value=0
  Divide : Product  Inputs=*/
  Trigonometric Function : Trigonometry  Operator=cos
  Trigonometric Function1 : Trigonometry
  Vector Concatenate : Concatenate  NumInputs=4
  Q_y : Outport
  wires:
  Vector Concatenate/1 -> Q_y/1
  Const/1 -> Divide/2
  Trigonometric Function/1 -> Vector Concatenate/1
  Const1/1 -> Vector Concatenate/2, Vector Concatenate/4
  Divide/1 -> Trigonometric Function1/1, Trigonometric Function/1
  h(Y Rad)/1 -> Divide/1
  Trigonometric Function1/1 -> Vector Concatenate/3

== system QuadSim/M3/B->M3 Quaternion/Z Quaternion ==
  Z Rad : Inport
  Const : Constant  Value=2
  Const1 : Constant  Value=0
  Divide : Product  Inputs=*/
  Trigonometric Function : Trigonometry  Operator=cos
  Trigonometric Function1 : Trigonometry
  Vector Concatenate : Concatenate  NumInputs=4
  Q_z : Outport
  wires:
  Vector Concatenate/1 -> Q_z/1
  Const/1 -> Divide/2
  Trigonometric Function/1 -> Vector Concatenate/1
  Const1/1 -> Vector Concatenate/3, Vector Concatenate/2
  Divide/1 -> Trigonometric Function1/1, Trigonometric Function/1
  Z Rad/1 -> Divide/1
  Trigonometric Function1/1 -> Vector Concatenate/4

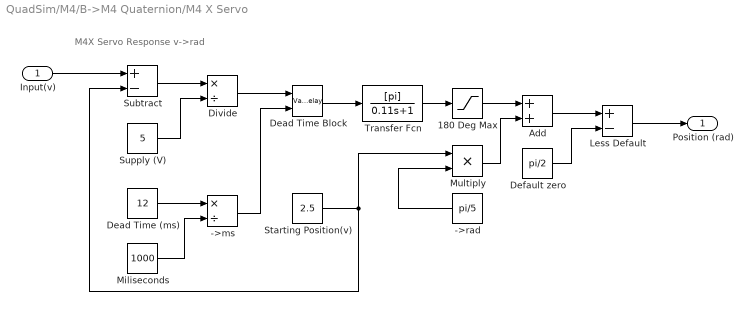
== system QuadSim/M4/B->M4 Quaternion/M4 X Servo  ==
  note: M4X Servo Response v->rad
  Input(v) : Inport
  ->ms : Product  Inputs=*/
  ->rad : Constant  Value=pi/5
  180 Deg Max : Saturate  UpperLimit=pi/2  LowerLimit=-pi/2
  Add : Sum
  Dead Time (ms) : Constant  Value=12
  Dead Time Block : VariableTransportDelay  MaximumDelay=10
  Default zero : Constant  Value=pi/2
  Divide : Product  Inputs=*/
  Less Default : Sum  Inputs=+-
  Miliseconds : Constant  Value=1000
  Multiply : Product  Inputs=**
  Starting Position(v) : Constant  Value=2.5
  Subtract : Sum  Inputs=+-
  Supply (V) : Constant  Value=5
  Transfer Fcn : TransferFcn  Numerator=[pi]  Denominator=[0.11 1]
  Position (rad) : Outport
  wires:
  Miliseconds/1 -> ->ms/2
  Dead Time (ms)/1 -> ->ms/1
  Default zero/1 -> Less Default/2
  Starting Position(v)/1 -> Multiply/1, Subtract/2
  Subtract/1 -> Divide/1
  Supply (V)/1 -> Divide/2
  Divide/1 -> Dead Time Block/1
  ->ms/1 -> Dead Time Block/2
  Dead Time Block/1 -> Transfer Fcn/1
  Transfer Fcn/1 -> 180 Deg Max/1
  180 Deg Max/1 -> Add/1
  ->rad/1 -> Multiply/2
  Multiply/1 -> Add/2
  Less Default/1 -> Position (rad)/1
  Add/1 -> Less Default/1
  Input(v)/1 -> Subtract/1

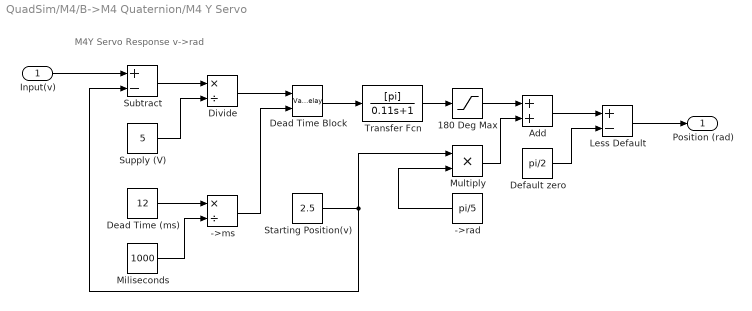
== system QuadSim/M4/B->M4 Quaternion/M4 Y Servo  ==
  note: M4Y Servo Response v->rad
  Input(v) : Inport
  ->ms : Product  Inputs=*/
  ->rad : Constant  Value=pi/5
  180 Deg Max : Saturate  UpperLimit=pi/2  LowerLimit=-pi/2
  Add : Sum
  Dead Time (ms) : Constant  Value=12
  Dead Time Block : VariableTransportDelay  MaximumDelay=10
  Default zero : Constant  Value=pi/2
  Divide : Product  Inputs=*/
  Less Default : Sum  Inputs=+-
  Miliseconds : Constant  Value=1000
  Multiply : Product  Inputs=**
  Starting Position(v) : Constant  Value=2.5
  Subtract : Sum  Inputs=+-
  Supply (V) : Constant  Value=5
  Transfer Fcn : TransferFcn  Numerator=[pi]  Denominator=[0.11 1]
  Position (rad) : Outport
  wires:
  Miliseconds/1 -> ->ms/2
  Dead Time (ms)/1 -> ->ms/1
  Default zero/1 -> Less Default/2
  Starting Position(v)/1 -> Multiply/1, Subtract/2
  Subtract/1 -> Divide/1
  Supply (V)/1 -> Divide/2
  Divide/1 -> Dead Time Block/1
  ->ms/1 -> Dead Time Block/2
  Dead Time Block/1 -> Transfer Fcn/1
  Transfer Fcn/1 -> 180 Deg Max/1
  180 Deg Max/1 -> Add/1
  ->rad/1 -> Multiply/2
  Multiply/1 -> Add/2
  Less Default/1 -> Position (rad)/1
  Add/1 -> Less Default/1
  Input(v)/1 -> Subtract/1
